simulink model "a7DOF"  (R2021a)
settings: Solver=VariableStepAuto  StartTime=0.0  StopTime=10.0  RelTol=1e-3
(part 2 of 2)

== system a7DOF/Type_Model/Magic_Model/Magic_Model_rl/Subsystem3 ==
  "Fz " : Inport
  Add : Sum  Inputs=+++
  Constant : Constant  Value=1.3
  Divide : Product  Inputs=/*
  Math Function : Math  Operator=square  SignedPower=on  SaturateOnIntegerOverflow=on
  Math Function1 : Math  Operator=square  SignedPower=on  SaturateOnIntegerOverflow=on
  Product : Product  RndMeth=Zero
  Sum : Sum  Inputs=|++
  Trigonometric Function : Trigonometry  Operator=atan
  Trigonometric Function1 : Trigonometry
  a1 : Gain  Gain=-22.1
  a2 : Gain  Gain=1011
  a3 : Gain  Gain=1078
  a4 : Gain  Gain=1.82
  a5 : Gain  Gain=0.208
  a6 : Gain  Gain=0
  a7 : Gain  Gain=-0.354
  a8 : Constant  Value=0.707
  "B " : Outport
  "E " : Outport  Port=2
  "D " : Outport  Port=3
  wires:
  Add/1 -> "E "/1
  a8/1 -> Add/3
  a7/1 -> Add/2
  a6/1 -> Add/1
  Math Function1/1 -> a6/1
  Divide/1 -> "B "/1
  a3/1 -> Divide/2
  Product/1 -> Divide/1
  Sum/1 -> Product/2, "D "/1
  Constant/1 -> Product/1
  Trigonometric Function1/1 -> a3/1
  a4/1 -> Trigonometric Function1/1
  Trigonometric Function/1 -> a4/1
  a5/1 -> Trigonometric Function/1
  a2/1 -> Sum/2
  a1/1 -> Sum/1
  Math Function/1 -> a1/1
  "Fz "/1 -> Math Function/1, a2/1, a5/1, Math Function1/1, a7/1

== system a7DOF/Type_Model/Magic_Model/Magic_Model_rr/Subsystem ==
  FZ : Inport
  Add : Sum
  Add1 : Sum
  Add2 : Sum  Inputs=+++
  B1 : Gain  Gain=-21.3
  B2 : Gain  Gain=1144
  B3 : Gain  Gain=49.6
  B4 : Gain  Gain=226
  B5 : Gain  Gain=0.069
  B6 : Gain  Gain=-0.006
  B7 : Gain  Gain=0.056
  "B8 " : Constant  Value=0.486
  C : Constant  Value=1.65
  Divide : Product  Inputs=/*
  Math Function : Math  Operator=square  SignedPower=on  SaturateOnIntegerOverflow=on
  Math Function1 : Math  SignedPower=on  SaturateOnIntegerOverflow=on
  Product : Product  RndMeth=Zero
  Product1 : Product  RndMeth=Zero
  "B " : Outport
  E : Outport  Port=2
  "D " : Outport  Port=3
  wires:
  Math Function/1 -> B1/1, B3/1, B6/1
  FZ/1 -> B2/1, Math Function/1, B7/1, B5/1, B4/1
  B1/1 -> Add/2
  Product1/1 -> Divide/1
  Add/1 -> Product1/1, "D "/1
  B2/1 -> Add/1
  B3/1 -> Add1/1
  B4/1 -> Add1/2
  B6/1 -> Add2/1
  Add2/1 -> E/1
  Divide/1 -> "B "/1
  B7/1 -> Add2/2
  B5/1 -> Math Function1/1
  Add1/1 -> Product/1
  Product/1 -> Divide/2
  "B8 "/1 -> Add2/3
  C/1 -> Product1/2
  Math Function1/1 -> Product/2

== system a7DOF/Type_Model/Magic_Model/Magic_Model_rr/Subsystem1 ==
  X : Inport
  B : Inport  Port=2
  E : Inport  Port=3
  D : Inport  Port=4
  Add2 : Sum
  Add3 : Sum  Inputs=+-
  Add4 : Sum  Inputs=+-
  C : Constant  Value=1.3
  Product{1..4} (4 alike) : Product  RndMeth=Zero
  Sh : Constant  Value=0
  Trigonometric Function1 : Trigonometry  Operator=atan
  Trigonometric Function2 : Trigonometry  Operator=atan
  Trigonometric Function3 : Trigonometry
  Fx0 : Outport
  wires:
  C/1 -> Product3/2
  Product3/1 -> Trigonometric Function3/1
  Product4/1 -> Fx0/1
  Trigonometric Function3/1 -> Product4/1
  D/1 -> Product4/2
  Product2/1 -> Add4/2
  Add2/1 -> Product1/2
  Add4/1 -> Trigonometric Function2/1
  B/1 -> Product1/1
  E/1 -> Product2/2
  Sh/1 -> Add2/2
  Product1/1 -> Add3/1, Add4/1, Trigonometric Function1/1
  Trigonometric Function1/1 -> Add3/2
  Add3/1 -> Product2/1
  Trigonometric Function2/1 -> Product3/1
  X/1 -> Add2/1

== system a7DOF/Type_Model/Magic_Model/Magic_Model_rr/Subsystem2 ==
  "X " : Inport
  B : Inport  Port=2
  E : Inport  Port=3
  D : Inport  Port=4
  Add3 : Sum  Inputs=+-
  Add4 : Sum  Inputs=+-
  C : Constant  Value=1.3
  Product{1..4} (4 alike) : Product  RndMeth=Zero
  Scope : Scope
  Trigonometric Function1 : Trigonometry  Operator=atan
  Trigonometric Function2 : Trigonometry  Operator=atan
  Trigonometric Function3 : Trigonometry
  Fy0 : Outport
  wires:
  C/1 -> Product3/2
  Product3/1 -> Trigonometric Function3/1
  Product4/1 -> Fy0/1
  Trigonometric Function3/1 -> Product4/1, Scope/1
  D/1 -> Product4/2
  Product2/1 -> Add4/2
  "X "/1 -> Product1/2
  Add4/1 -> Trigonometric Function2/1
  B/1 -> Product1/1
  E/1 -> Product2/2
  Product1/1 -> Add3/1, Add4/1, Trigonometric Function1/1
  Trigonometric Function1/1 -> Add3/2
  Add3/1 -> Product2/1
  Trigonometric Function2/1 -> Product3/1

== system a7DOF/Type_Model/Magic_Model/Magic_Model_rr/Subsystem3 ==
  "Fz " : Inport
  Add : Sum  Inputs=+++
  Constant : Constant  Value=1.3
  Divide : Product  Inputs=/*
  Math Function : Math  Operator=square  SignedPower=on  SaturateOnIntegerOverflow=on
  Math Function1 : Math  Operator=square  SignedPower=on  SaturateOnIntegerOverflow=on
  Product : Product  RndMeth=Zero
  Sum : Sum  Inputs=|++
  Trigonometric Function : Trigonometry  Operator=atan
  Trigonometric Function1 : Trigonometry
  a1 : Gain  Gain=-22.1
  a2 : Gain  Gain=1011
  a3 : Gain  Gain=1078
  a4 : Gain  Gain=1.82
  a5 : Gain  Gain=0.208
  a6 : Gain  Gain=0
  a7 : Gain  Gain=-0.354
  a8 : Constant  Value=0.707
  "B " : Outport
  "E " : Outport  Port=2
  "D " : Outport  Port=3
  wires:
  Add/1 -> "E "/1
  a8/1 -> Add/3
  a7/1 -> Add/2
  a6/1 -> Add/1
  Math Function1/1 -> a6/1
  Divide/1 -> "B "/1
  a3/1 -> Divide/2
  Product/1 -> Divide/1
  Sum/1 -> Product/2, "D "/1
  Constant/1 -> Product/1
  Trigonometric Function1/1 -> a3/1
  a4/1 -> Trigonometric Function1/1
  Trigonometric Function/1 -> a4/1
  a5/1 -> Trigonometric Function/1
  a2/1 -> Sum/2
  a1/1 -> Sum/1
  Math Function/1 -> a1/1
  "Fz "/1 -> Math Function/1, a2/1, a5/1, Math Function1/1, a7/1
